simulink model "LIN_F16Block"  (R2024b)
settings: Solver=ode5  StartTime=0.0  StopTime=20  FixedStep=0.001  RelTol=1e-3  EnableMultiTasking=on
model workspace (MAT data in the model file):
  x_a = [0 5 5.9 6 7 15]
undefined symbols (not defined in the file or in its folder): dLEF, fi_flag_Simulink, trim_control_lin, trim_state_lin, trim_thrust_lin
settings Model: Creator=keviczky  LastModifiedBy=quitu
settings SolverCC: AlgebraicLoopSolver=TrustRegion
settings DataIOCC: Decimation=50  SaveFormat=Array  SignalLoggingSaveFormat=ModelDataLogs  ReturnWorkspaceOutputs=off  SignalLoggingName=sigsOut
settings OptimizationCC: BooleanDataType=off  DefaultParameterBehavior=Inlined  BufferReuse=off
settings DebuggingCC: SaveWithParameterizedLinksMsg=none  UnderspecifiedInitializationDetection=Classic  MergeDetectMultiDrivingBlocksExec=none  SignalResolutionControl=TryResolveAllWithWarning  MultiTaskDSMMsg=warning  MultiTaskCondExecSysMsg=none  UnconnectedInputMsg=warning  UnconnectedOutputMsg=warning  UnconnectedLineMsg=warning  InitInArrayFormatMsg=none
settings HardwareCC: ProdBitPerPointer=32  ProdBitPerSizeT=32  ProdBitPerPtrDiffT=32  ProdLargestAtomicFloat=None  ProdIntDivRoundTo=Undefined  ProdEndianess=Unspecified  ProdWordSize=32  ProdHWDeviceType=32-bit Generic  TargetUnknown=on
settings ModelReferenceCC: EnableRefExpFcnMdlSchedulingChecks=on  PropagateSignalLabelsOutOfModel=off
settings RTWCC: GPUComputeCapability=3.5  DLArmComputeVersion=19.05
settings GRTTargetCC: CombineOutputUpdateFcns=off  GRTInterface=on
settings ConfigComp: CovMetricSettings=dw  CovSaveCumulativeToWorkspaceVar=on  CovSaveSingleToWorkspaceVar=on

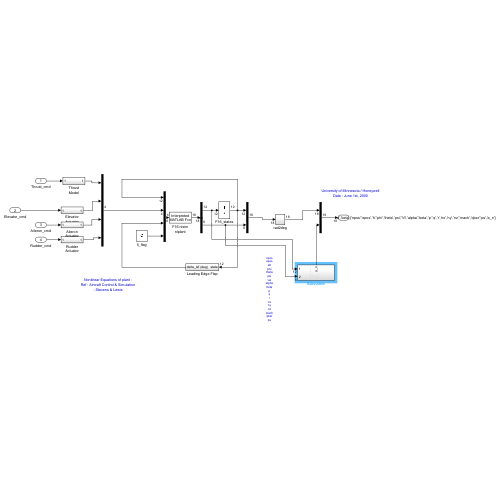
[thumbnail: Simulink's stored preview of the top-level diagram]
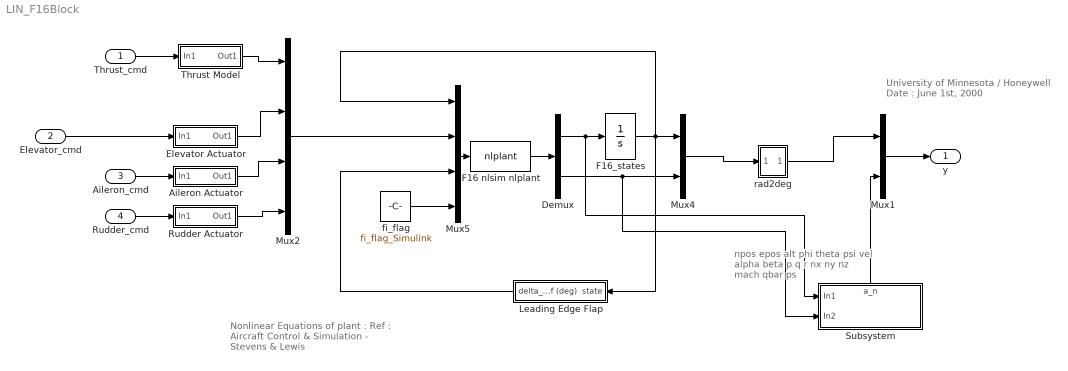
== system LIN_F16Block ==
  note: npos
      | epos
      | alt
      | phi
      | theta
      | psi
      | vel
      | alpha
      | beta
      | p
      | q
      | r
      | nx
      | ny
      | nz
      | mach
      | qbar
      | ps
  note: University of Minnesota / Honeywell
      | Date : June 1st, 2000
  note: Nonlinear Equations of plant :
      | Ref : Aircraft Control & Simulation
      | - Stevens & Lewis
  Thrust_cmd : Inport
  Elevator_cmd : Inport  Port=2
  Aileron_cmd : Inport  Port=3
  Rudder_cmd : Inport  Port=4
  Aileron Actuator : Subsystem  AncestorBlock=F16_Actuator_Library/Aileron Actuator
  Demux : Demux  Outputs=[12 6]
      settings: DisplayOption=none
  Elevator Actuator : Subsystem  AncestorBlock=F16_Actuator_Library/Elevator Actuator
  F16 nlsim nlplant : MATLABFcn  MATLABFcn=nlplant  OutputDimensions=18  OutputSignalType=real
  F16_states : Integrator  InitialCondition=trim_state_lin  ContinuousStateAttributes={'npos','epos','h','phi','theta','psi','Vt','alpha','beta','p','q','r'}
  Leading Edge Flap : Subsystem
  Mux1 : Mux  Inputs=2
  Mux2 : Mux
  Mux4 : Mux  Inputs=2
  Mux5 : Mux  Inputs=[12 4 1 1]
  Rudder Actuator : Subsystem  AncestorBlock=F16_Actuator_Library/Rudder Actuator
  Subsystem : Subsystem
      settings: PortSchema="{\"entries\":[{\"content\":{\"sides\":[{\"content\":{\"connectorIds\":[\"In1\",\"In2\"]},\"type\":\"ConnectorPlacement.EquallySpacedRectSide\",\"uuid\":\"0fa80532-1711-4d17-99de-7f3adea690f1\"},{\"content\":{\"side\":\"RIGHT\"},\"type\":\"ConnectorPlacement.EquallySpacedRectSide\",\"uuid\":\"88630073-4eeb-48de-8078-e73b8c0e76be\"},{\"content\":{\"connectorIds\":[\"Out1\"],\"side\":\"TOP\"},\"type\":\"ConnectorPlacement.EquallySpacedRectSide\",\"uuid\":\"dd9fce94-de3e-4405-9a79-87624e2de2b1\"}]},\"type\":\"ConnectorPlacement.EquallySpacedConnector\",\"uuid\":\"79c4658f-c6af-4489-959e-ff5bdee78491\"}],\"packageUris\":[\"http://schema.mathworks.com/mf0/Connector/R2020b\"],\"version\":\"1.0\"}"
  Thrust Model : Subsystem  AncestorBlock=F16_Actuator_Library/Thrust Model
  fi_flag : Constant  Value=fi_flag_Simulink
  rad2deg : Subsystem
  y : Outport  SignalName={'npos','epos','h','phi','theta','psi','Vt','alpha','beta','p','q','r','nx','ny','nz','mach','qbar','ps','a_n'}
  wires:
  Mux4/1 -> rad2deg/1(In1)
  F16 nlsim nlplant/1 -> Demux/1
  Demux/1 -> Subsystem/1(In1), F16_states/1
  Demux/2 -> Subsystem/2(In2), Mux4/2
  Mux5/1 -> F16 nlsim nlplant/1
  Mux2/1 -> Mux5/2
  F16_states/1 -> Mux5/1, Mux4/1, Leading Edge Flap/1(state)
  Thrust_cmd/1 -> Thrust Model/1(In1)
  Elevator_cmd/1 -> Elevator Actuator/1(In1)
  Aileron_cmd/1 -> Aileron Actuator/1(In1)
  Rudder_cmd/1 -> Rudder Actuator/1(In1)
  fi_flag/1 -> Mux5/4
  Leading Edge Flap/1(delta_lef (deg)) -> Mux5/3
  Elevator Actuator/1(Out1) -> Mux2/2
  Aileron Actuator/1(Out1) -> Mux2/3
  Rudder Actuator/1(Out1) -> Mux2/4
  Thrust Model/1(Out1) -> Mux2/1
  Mux1/1 -> y/1
  rad2deg/1(a_z) -> Mux1/1
  Subsystem/1(a_n) -> Mux1/2

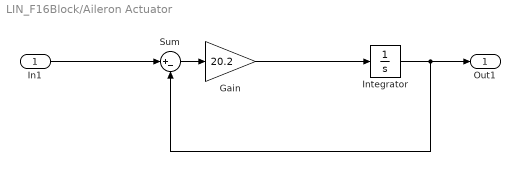
== system LIN_F16Block/Aileron Actuator ==
  In1 : Inport
  Gain : Gain  Gain=20.2  SaturateOnIntegerOverflow=on  OutDataTypeStr=Inherit: Same as input  ParamDataTypeStr=Inherit: Same as input
  "Integrator " : Integrator  InitialCondition=trim_control_lin(2)  UpperSaturationLimit=21.5  LowerSaturationLimit=-21.5  ContinuousStateAttributes='aileron_state'
  Sum : Sum  Inputs=|+-  InputSameDT=on  SaturateOnIntegerOverflow=on  OutDataTypeStr=Inherit: Same as first input
  Out1 : Outport
  wires:
  "Integrator "/1 -> Sum/2, Out1/1
  Gain/1 -> "Integrator "/1
  Sum/1 -> Gain/1
  In1/1 -> Sum/1

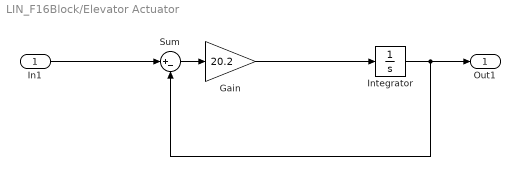
== system LIN_F16Block/Elevator Actuator ==
  In1 : Inport
  Gain : Gain  Gain=20.2  SaturateOnIntegerOverflow=on  OutDataTypeStr=Inherit: Same as input  ParamDataTypeStr=Inherit: Same as input
  "Integrator " : Integrator  InitialCondition=trim_control_lin(1)  UpperSaturationLimit=25  LowerSaturationLimit=-25  ContinuousStateAttributes='elevator_state'
  Sum : Sum  Inputs=|+-  InputSameDT=on  SaturateOnIntegerOverflow=on  OutDataTypeStr=Inherit: Same as first input
  Out1 : Outport
  wires:
  "Integrator "/1 -> Sum/2, Out1/1
  Gain/1 -> "Integrator "/1
  Sum/1 -> Gain/1
  In1/1 -> Sum/1

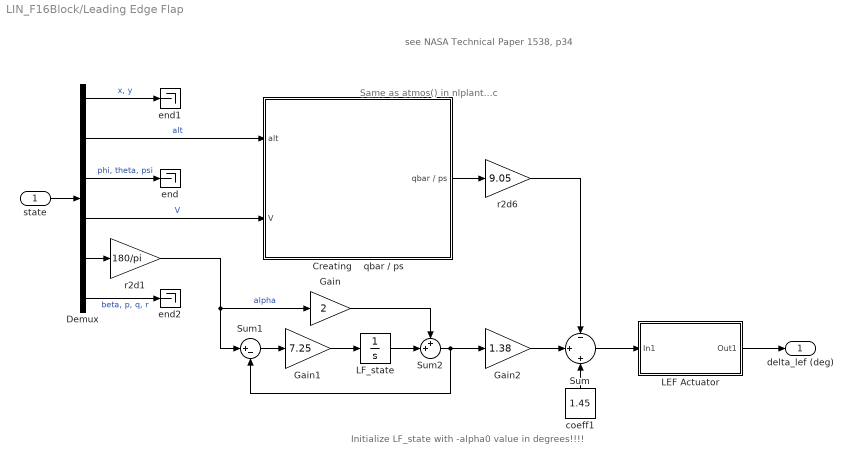
== system LIN_F16Block/Leading Edge Flap ==
  note: see NASA Technical Paper 1538, p34
  note: Same as atmos() in nlplant...c
  note: Initialize LF_state with -alpha0 value in degrees!!!!
  state : Inport
  Creating    qbar / ps : Subsystem
  Demux : Demux  Outputs=[2,1,3,1,1,4]
      settings: DisplayOption=none
  Gain : Gain  Gain=2  SaturateOnIntegerOverflow=on  OutDataTypeStr=Inherit: Same as input  ParamDataTypeStr=Inherit: Same as input
  Gain1 : Gain  Gain=7.25  SaturateOnIntegerOverflow=on  OutDataTypeStr=Inherit: Same as input  ParamDataTypeStr=Inherit: Same as input
  Gain2 : Gain  Gain=1.38  SaturateOnIntegerOverflow=on  OutDataTypeStr=Inherit: Same as input  ParamDataTypeStr=Inherit: Same as input
  LEF Actuator : Subsystem  AncestorBlock=F16_Actuator_Library/Aileron Actuator
  LF_state : Integrator  InitialCondition=-trim_state_lin(8)*180/pi
  Sum : Sum  Inputs=-|+|+  InputSameDT=on  SaturateOnIntegerOverflow=on  OutDataTypeStr=Inherit: Same as first input
  Sum1 : Sum  Inputs=|+-  InputSameDT=on  SaturateOnIntegerOverflow=on  OutDataTypeStr=Inherit: Same as first input
  Sum2 : Sum  Inputs=++|  InputSameDT=on  SaturateOnIntegerOverflow=on  OutDataTypeStr=Inherit: Same as first input
  coeff1 : Constant  Value=1.45
  end : Terminator
  end1 : Terminator
  end2 : Terminator
  r2d1 : Gain  Gain=180/pi  SaturateOnIntegerOverflow=on  OutDataTypeStr=Inherit: Same as input  ParamDataTypeStr=Inherit: Same as input
  r2d6 : Gain  Gain=9.05  SaturateOnIntegerOverflow=on  OutDataTypeStr=Inherit: Same as input  ParamDataTypeStr=Inherit: Same as input
  delta_lef (deg) : Outport
  wires:
  LEF Actuator/1(Out1) -> delta_lef (deg)/1
  Sum/1 -> LEF Actuator/1(In1)
  Demux/3 -> end/1  "phi, theta, psi"
  state/1 -> Demux/1
  Sum1/1 -> Gain1/1
  Gain1/1 -> LF_state/1
  Gain/1 -> Sum2/1
  Gain2/1 -> Sum/2
  Demux/1 -> end1/1  "x, y"
  Demux/5 -> r2d1/1
  Demux/6 -> end2/1  "beta, p, q, r"
  coeff1/1 -> Sum/3
  Sum2/1 -> Sum1/2, Gain2/1
  LF_state/1 -> Sum2/2
  r2d1/1 -> Sum1/1, Gain/1  "alpha"
  Demux/4 -> Creating    qbar / ps/2(V)  "V"
  Creating    qbar / ps/1(qbar / ps) -> r2d6/1
  r2d6/1 -> Sum/1
  Demux/2 -> Creating    qbar / ps/1(alt)  "alt"

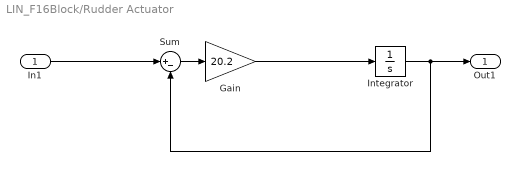
== system LIN_F16Block/Rudder Actuator ==
  In1 : Inport
  Gain : Gain  Gain=20.2  SaturateOnIntegerOverflow=on  OutDataTypeStr=Inherit: Same as input  ParamDataTypeStr=Inherit: Same as input
  "Integrator " : Integrator  InitialCondition=trim_control_lin(3)  UpperSaturationLimit=30  LowerSaturationLimit=-30  ContinuousStateAttributes='rudder_state'
  Sum : Sum  Inputs=|+-  InputSameDT=on  SaturateOnIntegerOverflow=on  OutDataTypeStr=Inherit: Same as first input
  Out1 : Outport
  wires:
  "Integrator "/1 -> Sum/2, Out1/1
  Gain/1 -> "Integrator "/1
  Sum/1 -> Gain/1
  In1/1 -> Sum/1

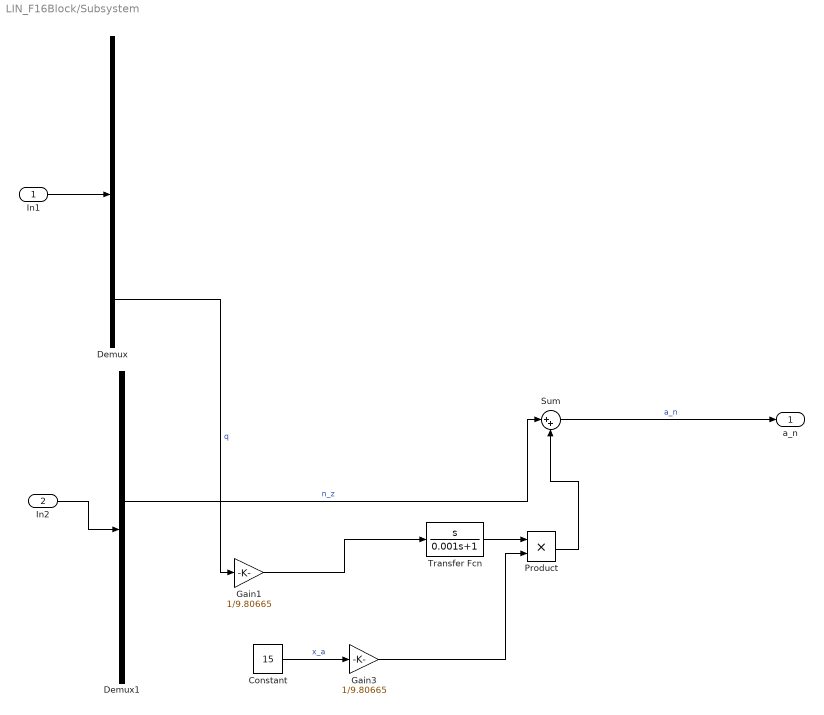
== system LIN_F16Block/Subsystem ==
  In1 : Inport
  In2 : Inport  Port=2
  Constant : Constant  Value=15
  Demux : Demux  Outputs=12
  Demux1 : Demux  Outputs=6
  Gain1 : Gain  Gain=1/9.80665
  Gain3 : Gain  Gain=1/9.80665
  Product : Product
  Sum : Sum  Inputs=|++
  Transfer Fcn : TransferFcn  Numerator=[1 0]  Denominator=[0.001 1]
  a_n : Outport
  wires:
  Sum/1 -> a_n/1  "a_n"
  Gain1/1 -> Transfer Fcn/1
  Transfer Fcn/1 -> Product/1
  Product/1 -> Sum/2
  Constant/1 -> Gain3/1  "x_a"
  Gain3/1 -> Product/2
  In1/1 -> Demux/1
  Demux/11 -> Gain1/1  "q"
  In2/1 -> Demux1/1
  Demux1/3 -> Sum/1  "n_z"

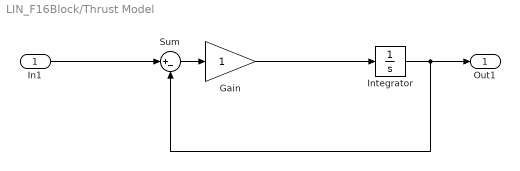
== system LIN_F16Block/Thrust Model ==
  In1 : Inport
  Gain : Gain  SaturateOnIntegerOverflow=on  OutDataTypeStr=Inherit: Same as input  ParamDataTypeStr=Inherit: Same as input
  "Integrator " : Integrator  InitialCondition=trim_thrust_lin  UpperSaturationLimit=30  LowerSaturationLimit=-30  ContinuousStateAttributes='thrust_state'
  Sum : Sum  Inputs=|+-  InputSameDT=on  SaturateOnIntegerOverflow=on  OutDataTypeStr=Inherit: Same as first input
  Out1 : Outport
  wires:
  "Integrator "/1 -> Sum/2, Out1/1
  Gain/1 -> "Integrator "/1
  Sum/1 -> Gain/1
  In1/1 -> Sum/1

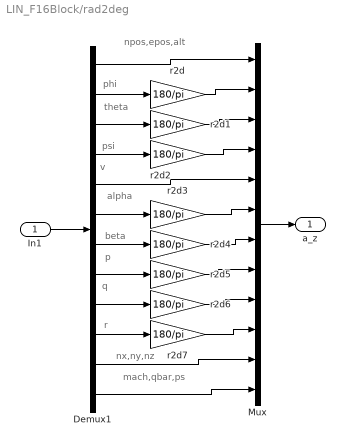
== system LIN_F16Block/rad2deg ==
  note: npos,epos,alt
  note: phi
  note: theta
  note: psi
  note: v
  note: alpha
  note: beta
  note: p
  note: q
  note: r
  note: nx,ny,nz
  note: mach,qbar,ps
  In1 : Inport
  Demux1 : Demux  Outputs=[3 1 1 1 1 1 1 1 1 1 3 3]
      settings: DisplayOption=none
  Mux : Mux  Inputs=[3 1 1 1 1 1 1 1 1 1 3 3]
  r2d{,1..7} (8 alike) : Gain  Gain=180/pi  SaturateOnIntegerOverflow=on  OutDataTypeStr=Inherit: Same as input  ParamDataTypeStr=Inherit: Same as input
  a_z : Outport
  wires:
  In1/1 -> Demux1/1
  Demux1/2 -> r2d/1
  Demux1/3 -> r2d1/1
  Demux1/4 -> r2d2/1
  Demux1/1 -> Mux/1
  Demux1/5 -> Mux/5
  r2d2/1 -> Mux/4
  r2d1/1 -> Mux/3
  r2d/1 -> Mux/2
  Demux1/6 -> r2d3/1
  Demux1/7 -> r2d4/1
  Demux1/8 -> r2d5/1
  Demux1/9 -> r2d6/1
  Demux1/10 -> r2d7/1
  r2d3/1 -> Mux/6
  r2d4/1 -> Mux/7
  r2d5/1 -> Mux/8
  r2d6/1 -> Mux/9
  r2d7/1 -> Mux/10
  Mux/1 -> a_z/1
  Demux1/11 -> Mux/11
  Demux1/12 -> Mux/12

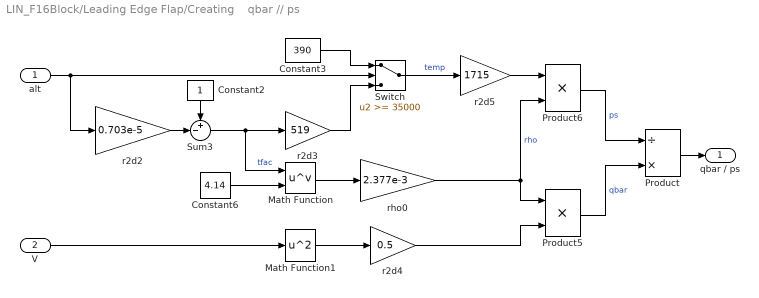
== system LIN_F16Block/Leading Edge Flap/Creating    qbar // ps ==
  alt : Inport
  V : Inport  Port=2
  Constant2 : Constant
  Constant3 : Constant  Value=390
  Constant6 : Constant  Value=4.14
  Math Function : Math  Operator=pow  SignedPower=on
  Math Function1 : Math  Operator=square  SignedPower=on
  Product : Product  Inputs=/*  InputSameDT=on  SaturateOnIntegerOverflow=on  OutDataTypeStr=Inherit: Same as first input
  Product5 : Product  Inputs=**  InputSameDT=on  SaturateOnIntegerOverflow=on  OutDataTypeStr=Inherit: Same as first input
  Product6 : Product  Inputs=**  InputSameDT=on  SaturateOnIntegerOverflow=on  OutDataTypeStr=Inherit: Same as first input
  Sum3 : Sum  Inputs=+-|  InputSameDT=on  SaturateOnIntegerOverflow=on  OutDataTypeStr=Inherit: Same as first input
  Switch : Switch  Threshold=35000
  r2d2 : Gain  Gain=0.703e-5  SaturateOnIntegerOverflow=on  OutDataTypeStr=Inherit: Same as input  ParamDataTypeStr=Inherit: Same as input
  r2d3 : Gain  Gain=519  SaturateOnIntegerOverflow=on  OutDataTypeStr=Inherit: Same as input  ParamDataTypeStr=Inherit: Same as input
  r2d4 : Gain  Gain=0.5  SaturateOnIntegerOverflow=on  OutDataTypeStr=Inherit: Same as input  ParamDataTypeStr=Inherit: Same as input
  r2d5 : Gain  Gain=1715  SaturateOnIntegerOverflow=on  OutDataTypeStr=Inherit: Same as input  ParamDataTypeStr=Inherit: Same as input
  rho0 : Gain  Gain=2.377e-3  SaturateOnIntegerOverflow=on  OutDataTypeStr=Inherit: Same as input  ParamDataTypeStr=Inherit: Same as input
  qbar / ps : Outport
  wires:
  alt/1 -> r2d2/1, Switch/2
  Sum3/1 -> Math Function/1, r2d3/1  "tfac"
  Constant3/1 -> Switch/1
  r2d3/1 -> Switch/3
  Constant6/1 -> Math Function/2
  rho0/1 -> Product5/1, Product6/2  "rho"
  Math Function1/1 -> r2d4/1
  r2d2/1 -> Sum3/2
  Constant2/1 -> Sum3/1
  Math Function/1 -> rho0/1
  r2d4/1 -> Product5/2
  Switch/1 -> r2d5/1  "temp"
  r2d5/1 -> Product6/1
  Product6/1 -> Product/1  "ps"
  Product5/1 -> Product/2  "qbar"
  Product/1 -> qbar / ps/1
  V/1 -> Math Function1/1

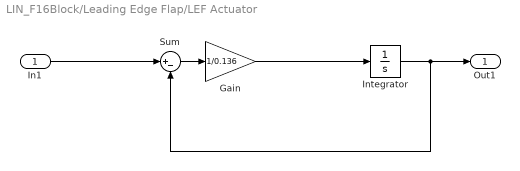
== system LIN_F16Block/Leading Edge Flap/LEF Actuator ==
  In1 : Inport
  Gain : Gain  Gain=1/0.136  SaturateOnIntegerOverflow=on  OutDataTypeStr=Inherit: Same as input  ParamDataTypeStr=Inherit: Same as input
  "Integrator " : Integrator  InitialCondition=dLEF  UpperSaturationLimit=21.5  LowerSaturationLimit=-21.5  ContinuousStateAttributes='LEF_actuator'
  Sum : Sum  Inputs=|+-  InputSameDT=on  SaturateOnIntegerOverflow=on  OutDataTypeStr=Inherit: Same as first input
  Out1 : Outport
  wires:
  "Integrator "/1 -> Sum/2, Out1/1
  Gain/1 -> "Integrator "/1
  Sum/1 -> Gain/1
  In1/1 -> Sum/1
